simulink model "NLModel_CornerBalance"  (R2016b)
settings: Solver=FixedStepAuto  StartTime=0.0  StopTime=5  FixedStep=0.0001  RelTol=1e-3
values from neighbouring files (symbols this model uses):
  C_psi = 3.1176e-5    (= 3.1176e-05)    [LQR_LQG_CornerDesign.m]
  g = 9.81    [LQR_LQG_CornerDesign.m]
  I_K_inv = inv(I_K)    [LQR_LQG_CornerDesign.m]
  I_R_inv = inv(I_R)    [LQR_LQG_CornerDesign.m]
  Kd = KKd * [eye(7), zeros(7,2)]*T_K    [LQR_LQG_CornerDesign.m]
  l_C = 0.066    [LQR_LQG_CornerDesign.m]
  m = 1.532    [LQR_LQG_CornerDesign.m]
  phi0 = [phi_10; phi_20+degtorad(-3); phi_30+degtorad(3)]    [LQR_LQG_CornerDesign.m]
  phi_20 = -2*atan(sqrt(2)-sqrt(3))    [LQR_LQG_CornerDesign.m]
  phi_30 = -pi/4    (= -0.785398163397)    [LQR_LQG_CornerDesign.m]
  Ta = 0.02    [LQR_LQG_CornerDesign.m]
  u_K0 = zeros(3,1)    [LQR_LQG_CornerDesign.m]
  u_R0 = zeros(3,1)    [LQR_LQG_CornerDesign.m]
  x_offset = [phi_offset; u_K_offset; u_R_offset]    [LQR_LQG_CornerDesign.m]
settings Model: Creator=michael  LastModifiedBy=michael

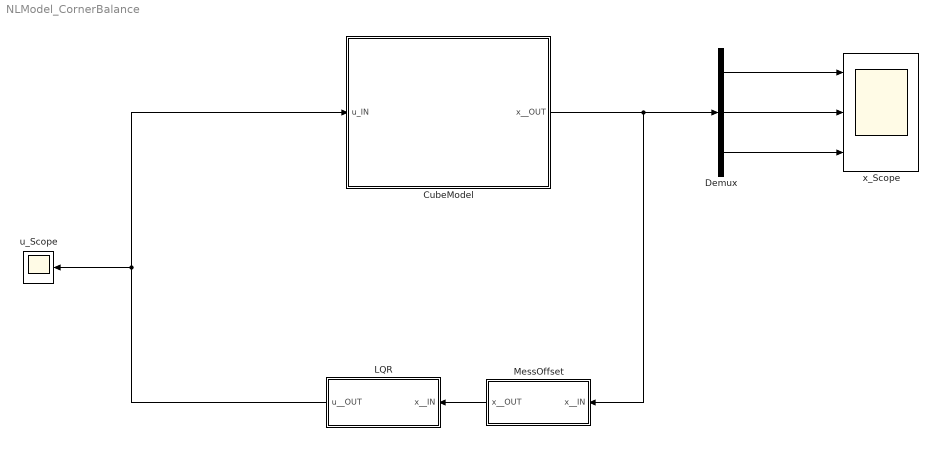
== system NLModel_CornerBalance ==
  CubeModel : Subsystem
  Demux : Demux  Outputs=3
  LQR : Subsystem
  MessOffset : Subsystem
  u_Scope : Scope
  x_Scope : Scope  NumInputPorts=3
  wires:
  Demux/1 -> x_Scope/1
  Demux/2 -> x_Scope/2
  Demux/3 -> x_Scope/3
  LQR/1(u__OUT) -> u_Scope/1, CubeModel/1(u_IN)
  CubeModel/1(x__OUT) -> MessOffset/1(x__IN), Demux/1
  MessOffset/1(x__OUT) -> LQR/1(x__IN)

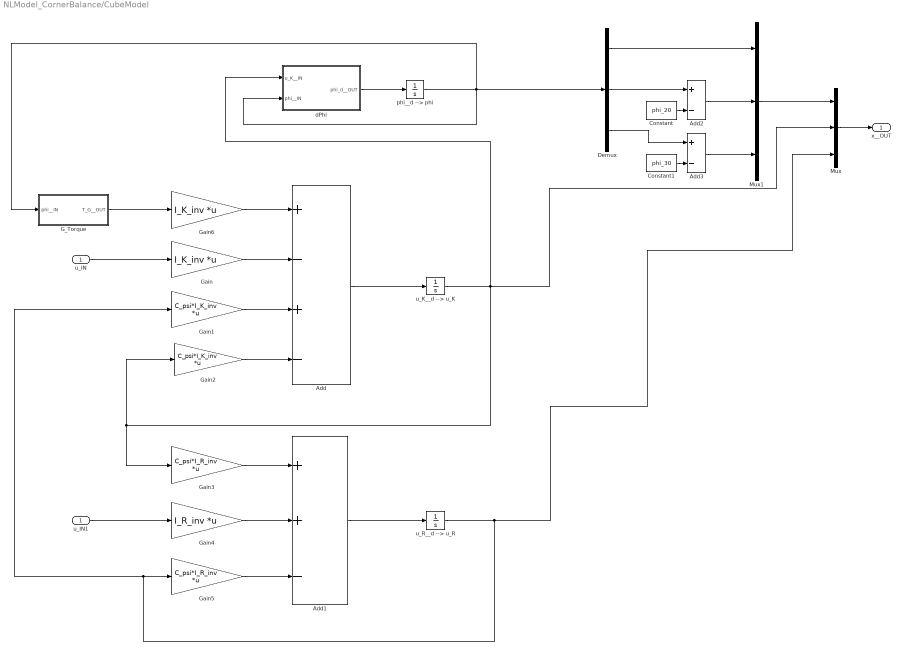
== system NLModel_CornerBalance/CubeModel ==
  u_IN : Inport
  Add : Sum  Inputs=+-+-
  Add1 : Sum  Inputs=++-
  Add2 : Sum  Inputs=+-
  Add3 : Sum  Inputs=+-
  Constant : Constant  Value=phi_20
  Constant1 : Constant  Value=phi_30
  Demux : Demux  Outputs=3
  G_Torque : Subsystem
  Gain : Gain  Gain=I_K_inv  Multiplication=Matrix(K*u) (u vector)
  Gain1 : Gain  Gain=C_psi*I_K_inv  Multiplication=Matrix(K*u) (u vector)
  Gain2 : Gain  Gain=C_psi*I_K_inv  Multiplication=Matrix(K*u) (u vector)
  Gain3 : Gain  Gain=C_psi*I_R_inv  Multiplication=Matrix(K*u) (u vector)
  Gain4 : Gain  Gain=I_R_inv  Multiplication=Matrix(K*u) (u vector)
  Gain5 : Gain  Gain=C_psi*I_R_inv  Multiplication=Matrix(K*u) (u vector)
  Gain6 : Gain  Gain=I_K_inv  Multiplication=Matrix(K*u)
  Mux : Mux  Inputs=3
  Mux1 : Mux  Inputs=3
  dPhi : Subsystem
  phi__d --> phi : Integrator  InitialCondition=phi0
  u_IN1 : InportShadow
  u_K__d --> u_K : Integrator  InitialCondition=u_K0
  u_R__d --> u_R : Integrator  InitialCondition=u_R0
  x__OUT : Outport
  wires:
  Add/1 -> u_K__d --> u_K/1
  G_Torque/1(T_G__OUT) -> Gain6/1
  Gain/1 -> Add/2
  u_IN/1 -> Gain/1
  Gain1/1 -> Add/3
  Gain2/1 -> Add/4
  u_K__d --> u_K/1 -> Gain3/1, Gain2/1, dPhi/1(u_K__IN), Mux/2
  Gain3/1 -> Add1/1
  Gain4/1 -> Add1/2
  u_IN1/1 -> Gain4/1
  Add1/1 -> u_R__d --> u_R/1
  Gain5/1 -> Add1/3
  u_R__d --> u_R/1 -> Mux/3, Gain5/1, Gain1/1
  dPhi/1(phi_d__OUT) -> phi__d --> phi/1
  Gain6/1 -> Add/1
  Mux/1 -> x__OUT/1
  phi__d --> phi/1 -> G_Torque/1(phi__IN), Demux/1, dPhi/2(phi__IN)
  Demux/2 -> Add2/1
  Demux/3 -> Add3/1
  Constant1/1 -> Add3/2
  Constant/1 -> Add2/2
  Demux/1 -> Mux1/1
  Add2/1 -> Mux1/2
  Add3/1 -> Mux1/3
  Mux1/1 -> Mux/1

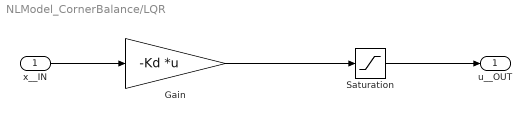
== system NLModel_CornerBalance/LQR ==
  x__IN : Inport  SampleTime=Ta
  Gain : Gain  Gain=-Kd  Multiplication=Matrix(K*u) (u vector)
  Saturation : Saturate  UpperLimit=0.11  LowerLimit=-0.11
  u__OUT : Outport
  wires:
  x__IN/1 -> Gain/1
  Gain/1 -> Saturation/1
  Saturation/1 -> u__OUT/1

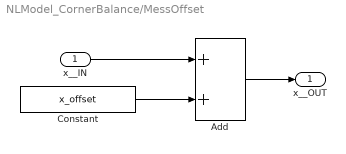
== system NLModel_CornerBalance/MessOffset ==
  x__IN : Inport
  Add : Sum
  Constant : Constant  Value=x_offset
  x__OUT : Outport
  wires:
  x__IN/1 -> Add/1
  Add/1 -> x__OUT/1
  Constant/1 -> Add/2

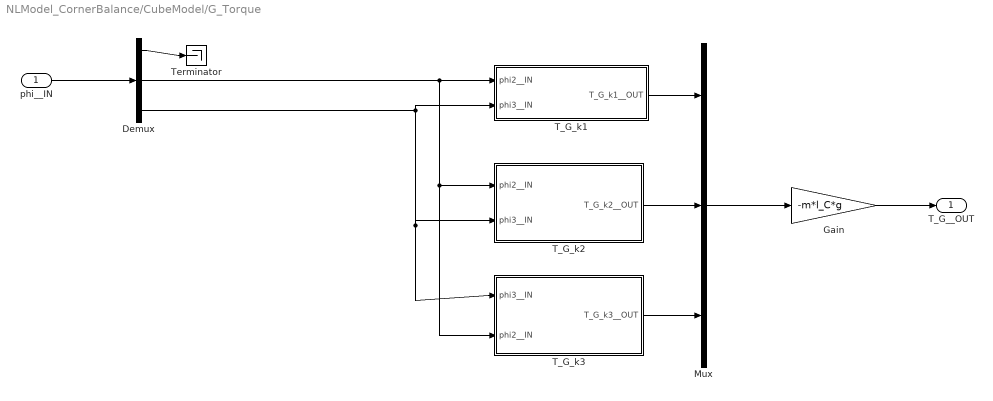
== system NLModel_CornerBalance/CubeModel/G_Torque ==
  phi__IN : Inport
  Demux : Demux  Outputs=3
  Gain : Gain  Gain=-m*l_C*g
  Mux : Mux  Inputs=3
  T_G_k1 : Subsystem
  T_G_k2 : Subsystem
  T_G_k3 : Subsystem
  Terminator : Terminator
  T_G__OUT : Outport
  wires:
  phi__IN/1 -> Demux/1
  Demux/1 -> Terminator/1
  Demux/2 -> T_G_k3/2(phi2__IN), T_G_k2/1(phi2__IN), T_G_k1/1(phi2__IN)
  Demux/3 -> T_G_k3/1(phi3__IN), T_G_k2/2(phi3__IN), T_G_k1/2(phi3__IN)
  T_G_k3/1(T_G_k3__OUT) -> Mux/3
  Mux/1 -> Gain/1
  T_G_k2/1(T_G_k2__OUT) -> Mux/2
  T_G_k1/1(T_G_k1__OUT) -> Mux/1
  Gain/1 -> T_G__OUT/1

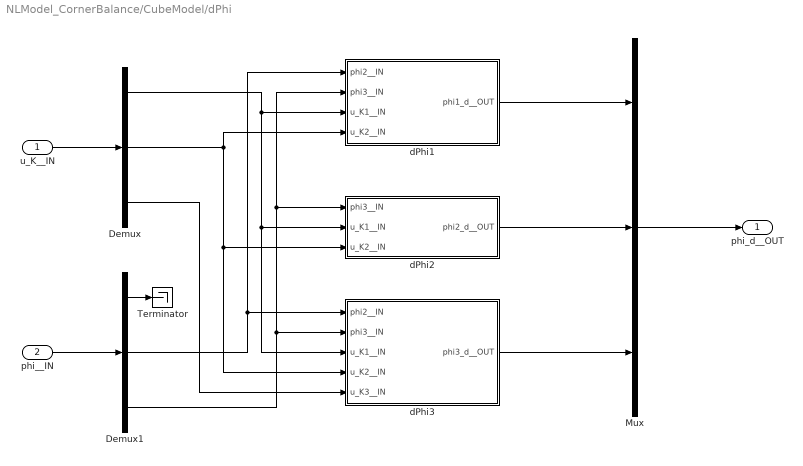
== system NLModel_CornerBalance/CubeModel/dPhi ==
  u_K__IN : Inport
  phi__IN : Inport  Port=2
  Demux : Demux  Outputs=3
  Demux1 : Demux  Outputs=3
  Mux : Mux  Inputs=3
  Terminator : Terminator
  dPhi1 : Subsystem
  dPhi2 : Subsystem
  dPhi3 : Subsystem
  phi_d__OUT : Outport
  wires:
  u_K__IN/1 -> Demux/1
  Mux/1 -> phi_d__OUT/1
  phi__IN/1 -> Demux1/1
  dPhi1/1(phi1_d__OUT) -> Mux/1
  dPhi2/1(phi2_d__OUT) -> Mux/2
  dPhi3/1(phi3_d__OUT) -> Mux/3
  Demux1/2 -> dPhi3/1(phi2__IN), dPhi1/1(phi2__IN)
  Demux1/3 -> dPhi3/2(phi3__IN), dPhi2/1(phi3__IN), dPhi1/2(phi3__IN)
  Demux1/1 -> Terminator/1
  Demux/2 -> dPhi2/3(u_K2__IN), dPhi3/4(u_K2__IN), dPhi1/4(u_K2__IN)
  Demux/3 -> dPhi3/5(u_K3__IN)
  Demux/1 -> dPhi1/3(u_K1__IN), dPhi2/2(u_K1__IN), dPhi3/3(u_K1__IN)

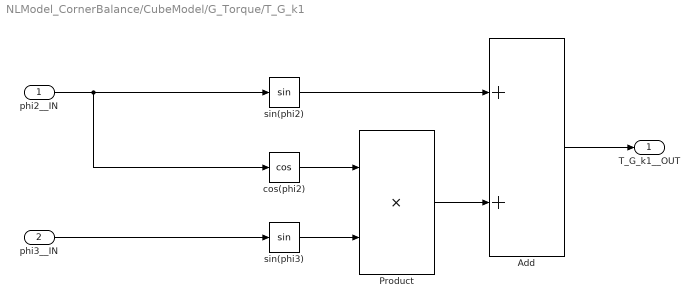
== system NLModel_CornerBalance/CubeModel/G_Torque/T_G_k1 ==
  phi2__IN : Inport
  phi3__IN : Inport  Port=2
  Add : Sum
  Product : Product
  cos(phi2) : Trigonometry  Operator=cos
  sin(phi2) : Trigonometry
  sin(phi3) : Trigonometry
  T_G_k1__OUT : Outport
  wires:
  phi2__IN/1 -> cos(phi2)/1, sin(phi2)/1
  cos(phi2)/1 -> Product/1
  sin(phi2)/1 -> Add/1
  Product/1 -> Add/2
  phi3__IN/1 -> sin(phi3)/1
  sin(phi3)/1 -> Product/2
  Add/1 -> T_G_k1__OUT/1

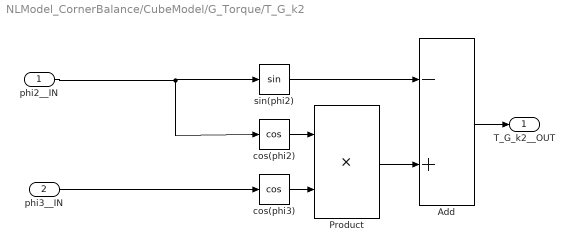
== system NLModel_CornerBalance/CubeModel/G_Torque/T_G_k2 ==
  phi2__IN : Inport
  phi3__IN : Inport  Port=2
  Add : Sum  Inputs=-+
  Product : Product
  cos(phi2) : Trigonometry  Operator=cos
  cos(phi3) : Trigonometry  Operator=cos
  sin(phi2) : Trigonometry
  T_G_k2__OUT : Outport
  wires:
  sin(phi2)/1 -> Add/1
  phi2__IN/1 -> cos(phi2)/1, sin(phi2)/1
  cos(phi2)/1 -> Product/1
  Add/1 -> T_G_k2__OUT/1
  phi3__IN/1 -> cos(phi3)/1
  cos(phi3)/1 -> Product/2
  Product/1 -> Add/2

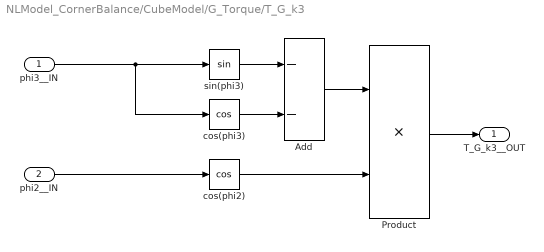
== system NLModel_CornerBalance/CubeModel/G_Torque/T_G_k3 ==
  phi3__IN : Inport
  phi2__IN : Inport  Port=2
  Add : Sum  Inputs=--
  Product : Product
  cos(phi2) : Trigonometry  Operator=cos
  cos(phi3) : Trigonometry  Operator=cos
  sin(phi3) : Trigonometry
  T_G_k3__OUT : Outport
  wires:
  Product/1 -> T_G_k3__OUT/1
  phi3__IN/1 -> cos(phi3)/1, sin(phi3)/1
  phi2__IN/1 -> cos(phi2)/1
  cos(phi3)/1 -> Add/2
  cos(phi2)/1 -> Product/2
  sin(phi3)/1 -> Add/1
  Add/1 -> Product/1

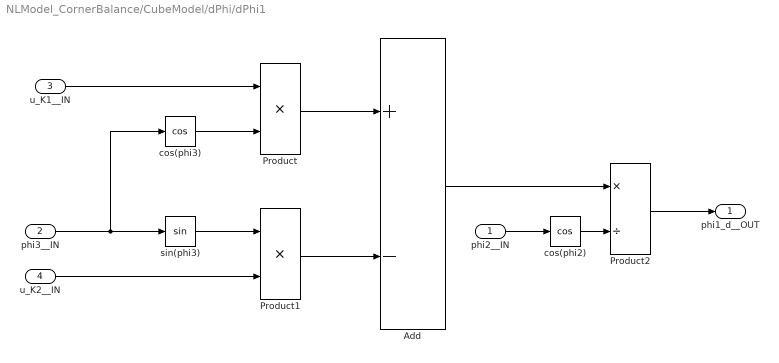
== system NLModel_CornerBalance/CubeModel/dPhi/dPhi1 ==
  phi2__IN : Inport
  phi3__IN : Inport  Port=2
  u_K1__IN : Inport  Port=3
  u_K2__IN : Inport  Port=4
  Add : Sum  Inputs=+-
  Product : Product  Inputs=**
  Product1 : Product  Inputs=**
  Product2 : Product  Inputs=*/
  cos(phi2) : Trigonometry  Operator=cos
  cos(phi3) : Trigonometry  Operator=cos
  sin(phi3) : Trigonometry
  phi1_d__OUT : Outport
  wires:
  phi3__IN/1 -> cos(phi3)/1, sin(phi3)/1
  cos(phi3)/1 -> Product/2
  u_K1__IN/1 -> Product/1
  sin(phi3)/1 -> Product1/1
  u_K2__IN/1 -> Product1/2
  Product/1 -> Add/1
  Product1/1 -> Add/2
  phi2__IN/1 -> cos(phi2)/1
  Add/1 -> Product2/1
  cos(phi2)/1 -> Product2/2
  Product2/1 -> phi1_d__OUT/1

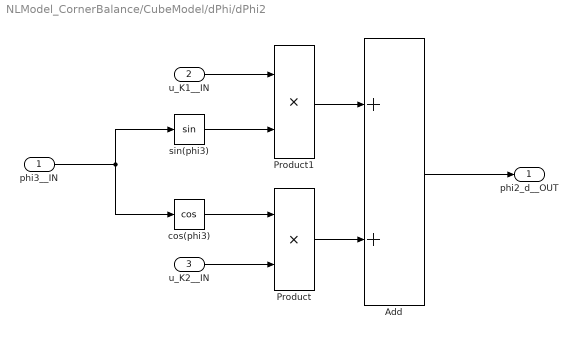
== system NLModel_CornerBalance/CubeModel/dPhi/dPhi2 ==
  phi3__IN : Inport
  u_K1__IN : Inport  Port=2
  u_K2__IN : Inport  Port=3
  Add : Sum
  Product : Product
  Product1 : Product
  cos(phi3) : Trigonometry  Operator=cos
  sin(phi3) : Trigonometry
  phi2_d__OUT : Outport
  wires:
  phi3__IN/1 -> sin(phi3)/1, cos(phi3)/1
  cos(phi3)/1 -> Product/1
  u_K2__IN/1 -> Product/2
  u_K1__IN/1 -> Product1/1
  sin(phi3)/1 -> Product1/2
  Product1/1 -> Add/1
  Product/1 -> Add/2
  Add/1 -> phi2_d__OUT/1

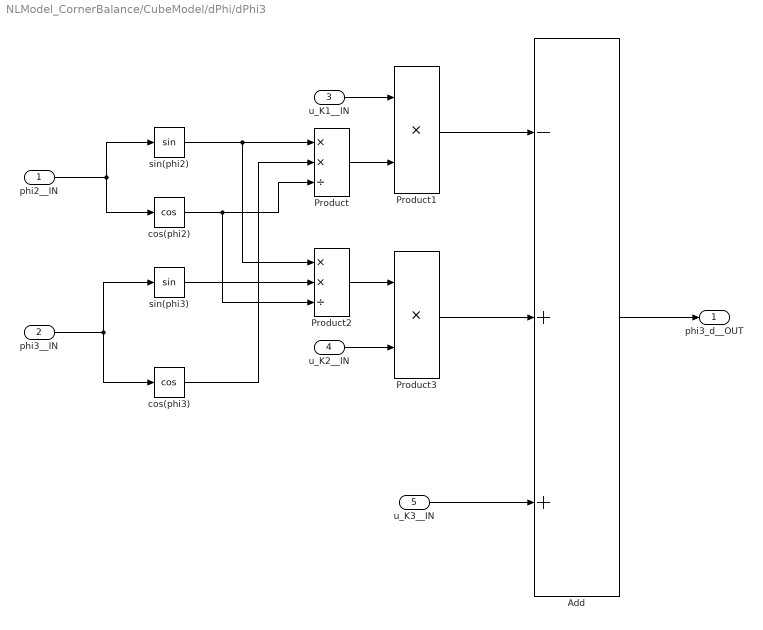
== system NLModel_CornerBalance/CubeModel/dPhi/dPhi3 ==
  phi2__IN : Inport
  phi3__IN : Inport  Port=2
  u_K1__IN : Inport  Port=3
  u_K2__IN : Inport  Port=4
  u_K3__IN : Inport  Port=5
  Add : Sum  Inputs=-++
  Product : Product  Inputs=**/
  Product1 : Product
  Product2 : Product  Inputs=**/
  Product3 : Product
  cos(phi2) : Trigonometry  Operator=cos
  cos(phi3) : Trigonometry  Operator=cos
  sin(phi2) : Trigonometry
  sin(phi3) : Trigonometry
  phi3_d__OUT : Outport
  wires:
  phi2__IN/1 -> cos(phi2)/1, sin(phi2)/1
  phi3__IN/1 -> cos(phi3)/1, sin(phi3)/1
  sin(phi2)/1 -> Product2/1, Product/1
  cos(phi3)/1 -> Product/2
  u_K1__IN/1 -> Product1/1
  Product/1 -> Product1/2
  cos(phi2)/1 -> Product2/3, Product/3
  sin(phi3)/1 -> Product2/2
  Product2/1 -> Product3/1
  u_K2__IN/1 -> Product3/2
  Product1/1 -> Add/1
  Product3/1 -> Add/2
  u_K3__IN/1 -> Add/3
  Add/1 -> phi3_d__OUT/1
